simulink model "a1_2_g1"  (R2023b)
settings: Solver=VariableStepAuto  StartTime=0.0  StopTime=5  RelTol=1e-3
settings Model: Creator=serkan  LastModifiedBy=serkan

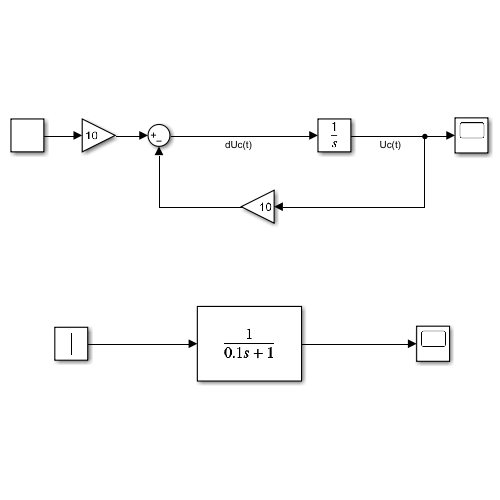
[thumbnail: Simulink's stored preview of the top-level diagram]
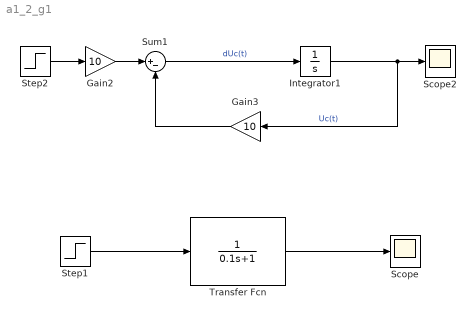
== system a1_2_g1 ==
  Gain2 : Gain  Gain=10
  Gain3 : Gain  Gain=10
  Integrator1 : Integrator
  Scope : Scope
  Scope2 : Scope
  Step1 : Step  SampleTime=0
  Step2 : Step  SampleTime=0
  Sum1 : Sum  Inputs=|+-
  Transfer Fcn : TransferFcn  Denominator=[0.1 1]
  wires:
  Step1/1 -> Transfer Fcn/1
  Transfer Fcn/1 -> Scope/1
  Gain2/1 -> Sum1/1
  Integrator1/1 -> Scope2/1, Gain3/1  "Uc(t)"
  Gain3/1 -> Sum1/2
  Step2/1 -> Gain2/1
  Sum1/1 -> Integrator1/1  "dUc(t)"
